simulink library "AEMS_Standard_Library"  (R2016b)
settings: Solver=ode45  StartTime=0.0  StopTime=10.0  RelTol=1e-3
undefined symbols (not defined in the file or in its folder): BkPY, carto, Cbx_extegr, Cbx_lpegrsys, Cbx_portegr, Cnx_bnk_nr_conf, Cnx_cyl_nr_conf, ConfigManagement, configuration_management, Cxx_dcm_io_tmr_end_xxxx, Cxx_dcm_rt_tmr_end, Cxx_DID_xxxx_IO_max, Cxx_DID_xxxx_IO_min, Cxx_egrhsofs, Cxx_vmaniegi, DEM_DEBOUNCE_FREEZE, DEM_DTR_CTL_INVISIBLE, DEM_DTR_CTL_NORMAL, Dem_DtrId2_XXX, Dem_DtrId3_XXX, Dem_DtrId4_XXX, Dem_DtrId5_XXX, Dem_DtrId6_XXX, Dem_DtrId7_XXX, Dem_DtrId8_XXX, Dem_DtrId9_XXX, Dem_DtrId_XXX, Dem_EnableConditionId2_XXX, Dem_EnableConditionId3_XXX, Dem_EnableConditionId4_XXX, Dem_EnableConditionId5_XXX, Dem_EnableConditionId6_XXX, Dem_EnableConditionId7_XXX, Dem_EnableConditionId8_XXX, Dem_EnableConditionId_XXX, Dem_EventId, Dem_EventId2_XXX, Dem_EventId3_XXX, Dem_EventId4_XXX, Dem_EventId5_XXX, Dem_EventId6_XXX, Dem_EventId7_XXX, Dem_EventId8_XXX, Dem_EventId9_XXX, Dem_EventId_Device_Faulttype, Dem_EventId_XXX, DEM_IUMPR_GENERAL_DENOMINATOR, DEM_OPCYC_IGNITION, Dem_RatioId2_XXX, Dem_RatioId3_XXX, Dem_RatioId4_XXX, Dem_RatioId5_XXX, Dem_RatioId6_XXX, Dem_RatioId7_XXX, Dem_RatioId8_XXX, Dem_RatioId_XXX, Dem_StorageConditionId2_XXX, Dem_StorageConditionId3_XXX, Dem_StorageConditionId4_XXX, Dem_StorageConditionId5_XXX ... (+65)
libraries: AEMS_Standard_Library x477, simulink x2
(part 15 of 39)

== system AEMS_Standard_Library/TIMER ==
  AEMS_SW_TIMER2 : Subsystem  Tag=[LIB]  mask(AEMS_SW_TIMER2){}
      mask help:
      | The block starts counter(Time) from zero when 'Start' input is
      | true and gets incremented in each time step with the 'Timestep'
      | value. The couter(Time) gets reset when 'Stop' becomes equal to true.
      settings: AttributesFormatString=%<MaskType>
      mask Help:
      | eval('path_lib=fileparts(which(''AEMS_Standard_Library''));');
      | doc_path = [path_lib '\help\AEMS_SW_TIMER2.pdf'];
      | eval('open(doc_path)')
      mask Display: disp(get_param(gcb,'name'));
  AEMS_SW_TIMER_INIT : Subsystem  Tag=[LIB]  mask(AEMS_SW_TIMER_INIT){}
      mask help: This block is a Software Timer. Increments the timer count with respect to given timestep. 'Init' input is to make the timer value initialized to 0.
      settings: AttributesFormatString=%<MaskType>
      mask Help:
      | eval('path_lib=fileparts(which(''AEMS_Standard_Library''));');
      | doc_path = [path_lib '\help\AEMS_SW_TIMER_INIT.pdf'];
      | eval('open(doc_path)')
      mask Display: disp('AEMS_SW_TIMER_INIT');
  AEMS_TIMER : Subsystem  Tag=[LIB]  mask(AEMS_TIMER){sample_time=0.01}
      mask prompts: sample_time "Clock :"
      mask help:
      | Timer
      |
      | I/O
      |  start_flag
      |    1 : timer count up
      |    0 : timer clear
      |  target_time
      |    Target time
      |
      |  alarm
      |    1 : timer_value >= target_time
      |    0 : timer_value < target_time
      |  timer_value
      |    Timer value(up count)
      mask init:
      | name=get_param(gcb,'MaskValueString');
      | sample_time=str2num(name);
      settings: AttributesFormatString="%<MaskType>\\nClock :  = %<sample_time>"
      mask Help:
      | eval('path_lib=fileparts(which(''AEMS_Standard_Library''));');
      | mskblk=get_param(gcbh,'MaskType');
      | doc_path = [path_lib '\help\',mskblk,'.pdf'];
      | eval('open(doc_path)');
      mask TypeOptions sample_time: 0.001 | 0.002 | 0.004 | 0.01 | 0.02 | 0.1
      mask Display: disp(sprintf('Clock = %s', char(name)))
  AEMS_TIMER1 : Subsystem  Tag=[LIB]  mask(AEMS_TIMER1){timeoutinit=0, initinit=0}
      mask prompts: timeoutinit "Timeout output initialisation"; initinit "Init input initialisation"
      mask help:
      | This block starts a timer and generates a timeout signal when the required duration has elapsed.The duration in seconds is set on edge rising init signal  and counting phase begins.Output timer gives the left time in seconds, that must pass before generating the timeout signal.If the init signal is true after the power supply, and if the timer must start, set init input initialisation to 0, else set it to 1.
      | If the timeout output must start at true, set timeout output initialisation to 1, else set it to 0.
      settings: AttributesFormatString=%<MaskType>\nTimeout output initialisation=%<timeoutinit>\nInit input initialisation=%<initinit>
      mask Help:
      | eval('path_lib=fileparts(which(''AEMS_Standard_Library''));');
      | doc_path = [path_lib '\help\AEMS_TIMER1.pdf'];
      | eval('open(doc_path)')
      mask Display:
      | plot([0.1 0.15 0.15 0.2 0.2 0.35],[0.67 0.67 0.9 0.9 0.67 0.67]);
      | plot([0.45 0.5 0.5 0.7 0.9],[0.05 0.05 0.3 0.05 0.05])
      | plot([0.45 0.7 0.7 0.9],[0.67 0.67 0.9 0.9])
  AEMS_TIMER_H : Subsystem  Tag=[LIB]  mask(AEMS_TIMER_H){sample_time=0.01}
      mask prompts: sample_time "Clock :"
      mask help:
      | Timer with holder
      |
      | I/O
      |  start_flag
      |    1 : timer count up
      |    0 : timer hold
      |  clear_flag
      |    1 : timer clear
      |    0 : None
      |  target_time
      |    Target time
      |
      |  alarm
      |    1 : timer_value >= target_time
      |    0 : timer_value < target_time
      |  timer_value
      |    Timer value(up count)
      mask init:
      | name=get_param(gcb,'MaskValueString');
      | sample_time=str2num(name);
      settings: AttributesFormatString="%<MaskType>\\nClock :  = %<sample_time>"
      mask Help:
      | eval('path_lib=fileparts(which(''AEMS_Standard_Library''));');
      | mskblk=get_param(gcbh,'MaskType');
      | doc_path = [path_lib '\help\',mskblk,'.pdf'];
      | eval('open(doc_path)');
      mask TypeOptions sample_time: 0.001 | 0.002 | 0.004 | 0.01 | 0.02 | 0.1
      mask Display: disp(sprintf('Clock = %s', char(name)))
  AEMS_TURN_OFF_DELAY : Subsystem  Tag=[LIB]  mask(AEMS_TURN_OFF_DELAY){timeoutinit=0, initinit=0}
      mask prompts: timeoutinit "Output initialization (0 or 1)"; initinit "Input initialization (0 or 1)"
      mask help:
      | When input is toggled from low to high, the output will respond immediately to the input by setting output low to high.
      | When input is toggled from high to low, the output will set from high to low after delaytime elapses.
      settings: AttributesFormatString=%<MaskType>\nOutput initialization=%<timeoutinit>\nInput initialization=%<initinit>
      mask Help:
      | eval('path_lib=fileparts(which(''AEMS_Standard_Library''));');
      | doc_path = [path_lib '\help\AEMS_TURN_OFF_DELAY.pdf'];
      | eval('open(doc_path)')
      mask Display: disp('AEMS_TURN_OFF_DELAY')
  AEMS_TURN_ON_DELAY : Subsystem  Tag=[LIB]  mask(AEMS_TURN_ON_DELAY){timeoutinit=0, initinit=0}
      mask prompts: timeoutinit "Output initialization (0 or 1)"; initinit "Input initialization (0 or 1)"
      mask help:
      | This block delays the output in rising edge state of output signal. The output (Out) is a boolean signal changes from 0 to 1 after the specified delay time.
      |
      | Initializations:
      | - Output initialization = beginning state of Output signal.
      | - Input initialization = state of Signal at -t used to determine the presence of a rising/falling edge at the first simulation step.
      settings: AttributesFormatString=%<MaskType>\nOutput initialization=%<timeoutinit>\nInput initialization=%<initinit>
      mask Help:
      | eval('path_lib=fileparts(which(''AEMS_Standard_Library''));');
      | doc_path = [path_lib '\help\AEMS_TURN_ON_DELAY.pdf'];
      | eval('open(doc_path)')
      mask Display:
      | plot([3 3.5 3.5 4 4 5 5 7.5 7.5 8.5], [5 5 6 6 5 5 6 6 5 5]);
      | plot([3 6.5 6.5 7.5 7.5 8.5], [2 2 3 3 2 2]);
      | plot([3 4.5], [5 6]);
      | plot([3 4.5], [6 5]);
      | text(5,0.4, 'Duration');
      | plot([5 6.5], [1 1]);
      | plot([5.2 5 5.2], [0.8 1 1.2]);
      | plot([6.3 6.5 6.3], [0.8 1 1.2]);
      | plot([5 5],[4.7 1.3]);
      | plot([6.5 6.5],[1.8 1.3]);
      | plot([7.5 7.5],[4.7 3.7]);
      | plot([0], [0]);
      | plot([8], [7]);

== system AEMS_Standard_Library/TRIGGER ==
  AEMS_EVENT : Subsystem  Tag=[LIB]  mask(AEMS_EVENT){sample_time=0.01, event_time=0.1}
      mask help:
      | Down edge event : Every Event_time
      |
      | * Can not use AEMS_EVENT library in triggered/enabled subsystem
      mask init:
      | name=get_param(gcb,'MaskValueString');
      | name=sprintf(strrep(name,'|','\n'));
      | name=strread(name,'%s','delimiter',',');
      settings: AttributesFormatString=%<MaskType>
      mask Help:
      | eval('path_lib=fileparts(which(''AEMS_Standard_Library''));');
      | mskblk=get_param(gcbh,'MaskType');
      | doc_path = [path_lib '\help\',mskblk,'.pdf'];
      | eval('open(doc_path)');
      mask Display: disp(sprintf('Sample_time = %s \nEvent_time = %s', char(name(1)) , char(name(2))))

== system AEMS_Standard_Library/BIT_OPERATION/AEMS_BITWISEAND ==
  In : Inport
  Mask : Inport  Port=2
  Chart : Stateflow chart
  Out : Outport
  wires:
  Chart/1(Out) -> Out/1
  Mask/1 -> Chart/2(Mask)
  In/1 -> Chart/1(Input_data)

== system AEMS_Standard_Library/BIT_OPERATION/AEMS_BITWISEOR ==
  In : Inport
  Mask : Inport  Port=2
  Chart : Stateflow chart
  Out : Outport
  wires:
  Chart/1(Out) -> Out/1
  Mask/1 -> Chart/2(Mask)
  In/1 -> Chart/1(Input_data)

== system AEMS_Standard_Library/BIT_OPERATION/AEMS_BITWISEXOR ==
  In : Inport
  Mask : Inport  Port=2
  Chart : Stateflow chart
  Out : Outport
  wires:
  In/1 -> Chart/1(Input_data)
  Mask/1 -> Chart/2(Mask)
  Chart/1(Out) -> Out/1

== system AEMS_Standard_Library/BIT_OPERATION/AEMS_BIT_GET ==
  In : Inport  Tag=AM,In,0,1,Name,C;CMP,Port,PortWidth,SampleTime;
  Bit_number : Inport  Tag=AM,In,0,1,Name,C;CMP,Port,PortWidth,SampleTime;  Port=2
  Chart : Stateflow chart  TreatAsAtomicUnit=on
  Bit_value : Outport  Tag=AM,Out,1,0,Name,NC;CMP,Port,OutputWhenDisabled,InitialOutput;
  wires:
  In/1 -> Chart/1(In)
  Chart/1(Bit_value) -> Bit_value/1
  Bit_number/1 -> Chart/2(Bit_number)

== system AEMS_Standard_Library/BIT_OPERATION/AEMS_BIT_SET16 ==
  Bit1 : Inport  Tag=AM,In,0,1,Name,C;CMP,Port,PortWidth,SampleTime;  OutDataTypeStr=boolean
  Bit2 : Inport  Tag=AM,In,0,1,Name,C;CMP,Port,PortWidth,SampleTime;  Port=2  OutDataTypeStr=boolean
  Bit3 : Inport  Tag=AM,In,0,1,Name,C;CMP,Port,PortWidth,SampleTime;  Port=3  OutDataTypeStr=boolean
  Bit4 : Inport  Tag=AM,In,0,1,Name,C;CMP,Port,PortWidth,SampleTime;  Port=4  OutDataTypeStr=boolean
  Bit5 : Inport  Tag=AM,In,0,1,Name,C;CMP,Port,PortWidth,SampleTime;  Port=5  OutDataTypeStr=boolean
  Bit6 : Inport  Tag=AM,In,0,1,Name,C;CMP,Port,PortWidth,SampleTime;  Port=6  OutDataTypeStr=boolean
  Bit7 : Inport  Tag=AM,In,0,1,Name,C;CMP,Port,PortWidth,SampleTime;  Port=7  OutDataTypeStr=boolean
  Bit8 : Inport  Tag=AM,In,0,1,Name,C;CMP,Port,PortWidth,SampleTime;  Port=8  OutDataTypeStr=boolean
  Bit9 : Inport  Tag=AM,In,0,1,Name,C;CMP,Port,PortWidth,SampleTime;  Port=9  OutDataTypeStr=boolean
  Bit10 : Inport  Tag=AM,In,0,1,Name,C;CMP,Port,PortWidth,SampleTime;  Port=10  OutDataTypeStr=boolean
  Bit11 : Inport  Tag=AM,In,0,1,Name,C;CMP,Port,PortWidth,SampleTime;  Port=11  OutDataTypeStr=boolean
  Bit12 : Inport  Tag=AM,In,0,1,Name,C;CMP,Port,PortWidth,SampleTime;  Port=12  OutDataTypeStr=boolean
  Bit13 : Inport  Tag=AM,In,0,1,Name,C;CMP,Port,PortWidth,SampleTime;  Port=13  OutDataTypeStr=boolean
  Bit14 : Inport  Tag=AM,In,0,1,Name,C;CMP,Port,PortWidth,SampleTime;  Port=14  OutDataTypeStr=boolean
  Bit15 : Inport  Tag=AM,In,0,1,Name,C;CMP,Port,PortWidth,SampleTime;  Port=15  OutDataTypeStr=boolean
  Bit16 : Inport  Tag=AM,In,0,1,Name,C;CMP,Port,PortWidth,SampleTime;  Port=16  OutDataTypeStr=boolean
  Chart : Stateflow chart  TreatAsAtomicUnit=on
  Out : Outport  Tag=AM,Out,1,0,Name,NC;CMP,Port,OutputWhenDisabled,InitialOutput;
  wires:
  Bit15/1 -> Chart/15(Bit15)
  Bit14/1 -> Chart/14(Bit14)
  Bit13/1 -> Chart/13(Bit13)
  Bit12/1 -> Chart/12(Bit12)
  Bit11/1 -> Chart/11(Bit11)
  Bit10/1 -> Chart/10(Bit10)
  Bit9/1 -> Chart/9(Bit9)
  Bit8/1 -> Chart/8(Bit8)
  Bit7/1 -> Chart/7(Bit7)
  Bit6/1 -> Chart/6(Bit6)
  Bit5/1 -> Chart/5(Bit5)
  Bit4/1 -> Chart/4(Bit4)
  Bit3/1 -> Chart/3(Bit3)
  Bit2/1 -> Chart/2(Bit2)
  Bit16/1 -> Chart/16(Bit16)
  Bit1/1 -> Chart/1(Bit1)
  Chart/1(Out) -> Out/1

== system AEMS_Standard_Library/BIT_OPERATION/AEMS_BIT_SET32 ==
  Bit1 : Inport  Tag=AM,In,0,1,Name,C;CMP,Port,PortWidth,SampleTime;  OutDataTypeStr=boolean
  Bit2 : Inport  Tag=AM,In,0,1,Name,C;CMP,Port,PortWidth,SampleTime;  Port=2  OutDataTypeStr=boolean
  Bit3 : Inport  Tag=AM,In,0,1,Name,C;CMP,Port,PortWidth,SampleTime;  Port=3  OutDataTypeStr=boolean
  Bit4 : Inport  Tag=AM,In,0,1,Name,C;CMP,Port,PortWidth,SampleTime;  Port=4  OutDataTypeStr=boolean
  Bit5 : Inport  Tag=AM,In,0,1,Name,C;CMP,Port,PortWidth,SampleTime;  Port=5  OutDataTypeStr=boolean
  Bit6 : Inport  Tag=AM,In,0,1,Name,C;CMP,Port,PortWidth,SampleTime;  Port=6  OutDataTypeStr=boolean
  Bit7 : Inport  Tag=AM,In,0,1,Name,C;CMP,Port,PortWidth,SampleTime;  Port=7  OutDataTypeStr=boolean
  Bit8 : Inport  Tag=AM,In,0,1,Name,C;CMP,Port,PortWidth,SampleTime;  Port=8  OutDataTypeStr=boolean
  Bit9 : Inport  Tag=AM,In,0,1,Name,C;CMP,Port,PortWidth,SampleTime;  Port=9  OutDataTypeStr=boolean
  Bit10 : Inport  Tag=AM,In,0,1,Name,C;CMP,Port,PortWidth,SampleTime;  Port=10  OutDataTypeStr=boolean
  Bit11 : Inport  Tag=AM,In,0,1,Name,C;CMP,Port,PortWidth,SampleTime;  Port=11  OutDataTypeStr=boolean
  Bit12 : Inport  Tag=AM,In,0,1,Name,C;CMP,Port,PortWidth,SampleTime;  Port=12  OutDataTypeStr=boolean
  Bit13 : Inport  Tag=AM,In,0,1,Name,C;CMP,Port,PortWidth,SampleTime;  Port=13  OutDataTypeStr=boolean
  Bit14 : Inport  Tag=AM,In,0,1,Name,C;CMP,Port,PortWidth,SampleTime;  Port=14  OutDataTypeStr=boolean
  Bit15 : Inport  Tag=AM,In,0,1,Name,C;CMP,Port,PortWidth,SampleTime;  Port=15  OutDataTypeStr=boolean
  Bit16 : Inport  Tag=AM,In,0,1,Name,C;CMP,Port,PortWidth,SampleTime;  Port=16  OutDataTypeStr=boolean
  Bit17 : Inport  Tag=AM,In,0,1,Name,C;CMP,Port,PortWidth,SampleTime;  Port=17  OutDataTypeStr=boolean
  Bit18 : Inport  Tag=AM,In,0,1,Name,C;CMP,Port,PortWidth,SampleTime;  Port=18  OutDataTypeStr=boolean
  Bit19 : Inport  Tag=AM,In,0,1,Name,C;CMP,Port,PortWidth,SampleTime;  Port=19  OutDataTypeStr=boolean
  Bit20 : Inport  Tag=AM,In,0,1,Name,C;CMP,Port,PortWidth,SampleTime;  Port=20  OutDataTypeStr=boolean
  Bit21 : Inport  Tag=AM,In,0,1,Name,C;CMP,Port,PortWidth,SampleTime;  Port=21  OutDataTypeStr=boolean
  Bit22 : Inport  Tag=AM,In,0,1,Name,C;CMP,Port,PortWidth,SampleTime;  Port=22  OutDataTypeStr=boolean
  Bit23 : Inport  Tag=AM,In,0,1,Name,C;CMP,Port,PortWidth,SampleTime;  Port=23  OutDataTypeStr=boolean
  Bit24 : Inport  Tag=AM,In,0,1,Name,C;CMP,Port,PortWidth,SampleTime;  Port=24  OutDataTypeStr=boolean
  Bit25 : Inport  Tag=AM,In,0,1,Name,C;CMP,Port,PortWidth,SampleTime;  Port=25  OutDataTypeStr=boolean
  Bit26 : Inport  Tag=AM,In,0,1,Name,C;CMP,Port,PortWidth,SampleTime;  Port=26  OutDataTypeStr=boolean
  Bit27 : Inport  Tag=AM,In,0,1,Name,C;CMP,Port,PortWidth,SampleTime;  Port=27  OutDataTypeStr=boolean
  Bit28 : Inport  Tag=AM,In,0,1,Name,C;CMP,Port,PortWidth,SampleTime;  Port=28  OutDataTypeStr=boolean
  Bit29 : Inport  Tag=AM,In,0,1,Name,C;CMP,Port,PortWidth,SampleTime;  Port=29  OutDataTypeStr=boolean
  Bit30 : Inport  Tag=AM,In,0,1,Name,C;CMP,Port,PortWidth,SampleTime;  Port=30  OutDataTypeStr=boolean
  Bit31 : Inport  Tag=AM,In,0,1,Name,C;CMP,Port,PortWidth,SampleTime;  Port=31  OutDataTypeStr=boolean
  Bit32 : Inport  Tag=AM,In,0,1,Name,C;CMP,Port,PortWidth,SampleTime;  Port=32  OutDataTypeStr=boolean
  Chart : Stateflow chart  TreatAsAtomicUnit=on
  Out : Outport  Tag=AM,Out,1,0,Name,NC;CMP,Port,OutputWhenDisabled,InitialOutput;  OutDataTypeStr=uint32
  wires:
  Bit15/1 -> Chart/15(Bit15)
  Bit14/1 -> Chart/14(Bit14)
  Bit13/1 -> Chart/13(Bit13)
  Bit12/1 -> Chart/12(Bit12)
  Bit11/1 -> Chart/11(Bit11)
  Bit10/1 -> Chart/10(Bit10)
  Bit9/1 -> Chart/9(Bit9)
  Bit8/1 -> Chart/8(Bit8)
  Bit7/1 -> Chart/7(Bit7)
  Bit6/1 -> Chart/6(Bit6)
  Bit5/1 -> Chart/5(Bit5)
  Bit4/1 -> Chart/4(Bit4)
  Bit3/1 -> Chart/3(Bit3)
  Bit2/1 -> Chart/2(Bit2)
  Bit16/1 -> Chart/16(Bit16)
  Bit1/1 -> Chart/1(Bit1)
  Chart/1(Out) -> Out/1
  Bit17/1 -> Chart/17(Bit17)
  Bit22/1 -> Chart/22(Bit22)
  Bit21/1 -> Chart/21(Bit21)
  Bit24/1 -> Chart/24(Bit24)
  Bit19/1 -> Chart/19(Bit19)
  Bit20/1 -> Chart/20(Bit20)
  Bit23/1 -> Chart/23(Bit23)
  Bit18/1 -> Chart/18(Bit18)
  Bit25/1 -> Chart/25(Bit25)
  Bit26/1 -> Chart/26(Bit26)
  Bit27/1 -> Chart/27(Bit27)
  Bit28/1 -> Chart/28(Bit28)
  Bit29/1 -> Chart/29(Bit29)
  Bit30/1 -> Chart/30(Bit30)
  Bit31/1 -> Chart/31(Bit31)
  Bit32/1 -> Chart/32(Bit32)

== system AEMS_Standard_Library/BIT_OPERATION/AEMS_BIT_SET8 ==
  Bit1 : Inport  Tag=AM,In,0,1,Name,C;CMP,Port,PortWidth,SampleTime;
  Bit2 : Inport  Tag=AM,In,0,1,Name,C;CMP,Port,PortWidth,SampleTime;  Port=2
  Bit3 : Inport  Tag=AM,In,0,1,Name,C;CMP,Port,PortWidth,SampleTime;  Port=3
  Bit4 : Inport  Tag=AM,In,0,1,Name,C;CMP,Port,PortWidth,SampleTime;  Port=4
  Bit5 : Inport  Tag=AM,In,0,1,Name,C;CMP,Port,PortWidth,SampleTime;  Port=5
  Bit6 : Inport  Tag=AM,In,0,1,Name,C;CMP,Port,PortWidth,SampleTime;  Port=6
  Bit7 : Inport  Tag=AM,In,0,1,Name,C;CMP,Port,PortWidth,SampleTime;  Port=7
  Bit8 : Inport  Tag=AM,In,0,1,Name,C;CMP,Port,PortWidth,SampleTime;  Port=8
  Chart : Stateflow chart  TreatAsAtomicUnit=on
  Out : Outport  Tag=AM,Out,1,0,Name,NC;CMP,Port,OutputWhenDisabled,InitialOutput;
  wires:
  Bit8/1 -> Chart/8(Bit8)
  Bit7/1 -> Chart/7(Bit7)
  Bit6/1 -> Chart/6(Bit6)
  Bit5/1 -> Chart/5(Bit5)
  Bit4/1 -> Chart/4(Bit4)
  Bit3/1 -> Chart/3(Bit3)
  Bit2/1 -> Chart/2(Bit2)
  Bit1/1 -> Chart/1(Bit1)
  Chart/1(Out) -> Out/1

== system AEMS_Standard_Library/BIT_OPERATION/AEMS_CONVERT_1BYTE_TO_2BYTE ==
  in_1byte_first : Inport  PortDimensions=1
      settings: AttributesFormatString=<tsample=%<SampleTime>>
  in_1byte_second : Inport  Port=2  PortDimensions=1
      settings: AttributesFormatString=<tsample=%<SampleTime>>
  AEMS_CONVERT_1BYTE_TO_8BIT : AEMS_Standard_Library/BIT_OPERATION/AEMS_CONVERT_1BYTE_TO_8BIT  Tag=[LIB]
  AEMS_CONVERT_1BYTE_TO_8BIT1 : AEMS_Standard_Library/BIT_OPERATION/AEMS_CONVERT_1BYTE_TO_8BIT  Tag=[LIB]
  CONVERT_16BIT_TO_2BYTE : Subsystem
  out_2byte : Outport
  wires:
  CONVERT_16BIT_TO_2BYTE/1(out_2byte) -> out_2byte/1  "out_2byte"
  in_1byte_second/1 -> AEMS_CONVERT_1BYTE_TO_8BIT/1  "in_1byte_second"
  in_1byte_first/1 -> AEMS_CONVERT_1BYTE_TO_8BIT1/1  "in_1byte_first"
  AEMS_CONVERT_1BYTE_TO_8BIT/8 -> CONVERT_16BIT_TO_2BYTE/16(bit15)
  AEMS_CONVERT_1BYTE_TO_8BIT/7 -> CONVERT_16BIT_TO_2BYTE/15(bit14)
  AEMS_CONVERT_1BYTE_TO_8BIT/6 -> CONVERT_16BIT_TO_2BYTE/14(bit13)
  AEMS_CONVERT_1BYTE_TO_8BIT/5 -> CONVERT_16BIT_TO_2BYTE/13(bit12)
  AEMS_CONVERT_1BYTE_TO_8BIT/4 -> CONVERT_16BIT_TO_2BYTE/12(bit11)
  AEMS_CONVERT_1BYTE_TO_8BIT/3 -> CONVERT_16BIT_TO_2BYTE/11(bit10)
  AEMS_CONVERT_1BYTE_TO_8BIT/2 -> CONVERT_16BIT_TO_2BYTE/10(bit9)
  AEMS_CONVERT_1BYTE_TO_8BIT/1 -> CONVERT_16BIT_TO_2BYTE/9(bit8)
  AEMS_CONVERT_1BYTE_TO_8BIT1/8 -> CONVERT_16BIT_TO_2BYTE/8(bit7)
  AEMS_CONVERT_1BYTE_TO_8BIT1/7 -> CONVERT_16BIT_TO_2BYTE/7(bit6)
  AEMS_CONVERT_1BYTE_TO_8BIT1/6 -> CONVERT_16BIT_TO_2BYTE/6(bit5)
  AEMS_CONVERT_1BYTE_TO_8BIT1/5 -> CONVERT_16BIT_TO_2BYTE/5(bit4)
  AEMS_CONVERT_1BYTE_TO_8BIT1/4 -> CONVERT_16BIT_TO_2BYTE/4(bit3)
  AEMS_CONVERT_1BYTE_TO_8BIT1/3 -> CONVERT_16BIT_TO_2BYTE/3(bit2)
  AEMS_CONVERT_1BYTE_TO_8BIT1/2 -> CONVERT_16BIT_TO_2BYTE/2(bit1)
  AEMS_CONVERT_1BYTE_TO_8BIT1/1 -> CONVERT_16BIT_TO_2BYTE/1(bit0)

== system AEMS_Standard_Library/BIT_OPERATION/AEMS_CONVERT_1BYTE_TO_8BIT ==
  in_1byte : Inport  OutDataTypeStr=uint8  PortDimensions=1
      settings: AttributesFormatString=<tsample=%<SampleTime>>
  Constant : Constant  Value=128  OutDataTypeStr=uint8
  Constant1 : Constant  Value=64  OutDataTypeStr=uint8
  Constant2 : Constant  Value=32  OutDataTypeStr=uint8
  Constant3 : Constant  Value=16  OutDataTypeStr=uint8
  Constant4 : Constant  Value=8  OutDataTypeStr=uint8
  Constant5 : Constant  Value=4  OutDataTypeStr=uint8
  Constant6 : Constant  Value=2  OutDataTypeStr=uint8
  Constant7 : Constant  OutDataTypeStr=uint8
  Relational Operator{,1..7} (8 alike) : RelationalOperator  OutDataTypeStr=boolean  RndMeth=Nearest  InputSameDT=on
  Sum{,1..6} (7 alike) : Sum  Inputs=-+  SaturateOnIntegerOverflow=on  InputSameDT=on
  Switch{,1..6} (7 alike) : Switch  Threshold=0.5  SaturateOnIntegerOverflow=on  InputSameDT=on
  bit0 : Outport
  bit1 : Outport  Port=2
  bit2 : Outport  Port=3
  bit3 : Outport  Port=4
  bit4 : Outport  Port=5
  bit5 : Outport  Port=6
  bit6 : Outport  Port=7
  bit7 : Outport  Port=8
  wires:
  Relational Operator7/1 -> bit0/1  "bit0"
  Switch6/1 -> Relational Operator7/1
  Constant7/1 -> Relational Operator7/2
  Switch5/1 -> Switch6/3, Sum6/2, Relational Operator6/1
  Relational Operator6/1 -> bit1/1, Switch6/2  "bit1"
  Sum6/1 -> Switch6/1
  Constant6/1 -> Relational Operator6/2, Sum6/1
  Switch4/1 -> Switch5/3, Sum5/2, Relational Operator5/1
  Relational Operator5/1 -> Switch5/2, bit2/1  "bit2"
  Sum5/1 -> Switch5/1
  Constant5/1 -> Sum5/1, Relational Operator5/2
  Switch3/1 -> Sum4/2, Switch4/3, Relational Operator4/1
  Relational Operator4/1 -> bit3/1, Switch4/2  "bit3"
  Sum4/1 -> Switch4/1
  Constant4/1 -> Relational Operator4/2, Sum4/1
  Switch2/1 -> Switch3/3, Sum3/2, Relational Operator3/1
  Relational Operator3/1 -> Switch3/2, bit4/1  "bit4"
  Sum3/1 -> Switch3/1
  Constant3/1 -> Sum3/1, Relational Operator3/2
  Switch1/1 -> Switch2/3, Sum2/2, Relational Operator2/1
  Relational Operator2/1 -> bit5/1, Switch2/2  "bit5"
  Sum2/1 -> Switch2/1
  Constant2/1 -> Relational Operator2/2, Sum2/1
  Relational Operator1/1 -> Switch1/2, bit6/1  "bit6"
  Sum1/1 -> Switch1/1
  Switch/1 -> Switch1/3, Sum1/2, Relational Operator1/1
  Constant1/1 -> Sum1/1, Relational Operator1/2
  Sum/1 -> Switch/1
  Relational Operator/1 -> Switch/2, bit7/1  "bit7"
  Constant/1 -> Sum/1, Relational Operator/2
  in_1byte/1 -> Switch/3, Sum/2, Relational Operator/1  "in_1byte"

== system AEMS_Standard_Library/BIT_OPERATION/AEMS_CONVERT_2BYTE_TO_1BYTE ==
  in_2byte : Inport  OutDataTypeStr=uint16  PortDimensions=1
      settings: AttributesFormatString=<tsample=%<SampleTime>>
  AEMS_CONVERT_8BIT_TO_1BYTE : AEMS_Standard_Library/BIT_OPERATION/AEMS_CONVERT_8BIT_TO_1BYTE  Tag=[LIB]
  AEMS_CONVERT_8BIT_TO_1BYTE1 : AEMS_Standard_Library/BIT_OPERATION/AEMS_CONVERT_8BIT_TO_1BYTE  Tag=[LIB]
  CONVERT_2BYTE_TO_16BIT : Subsystem
  out_1byte_first : Outport
  out_1byte_second : Outport  Port=2
  wires:
  AEMS_CONVERT_8BIT_TO_1BYTE/1 -> out_1byte_second/1  "out_1byte_second"
  AEMS_CONVERT_8BIT_TO_1BYTE1/1 -> out_1byte_first/1  "out_1byte_first"
  in_2byte/1 -> CONVERT_2BYTE_TO_16BIT/1(in_2byte)  "in_2byte"
  CONVERT_2BYTE_TO_16BIT/16(bit15) -> AEMS_CONVERT_8BIT_TO_1BYTE/8
  CONVERT_2BYTE_TO_16BIT/15(bit14) -> AEMS_CONVERT_8BIT_TO_1BYTE/7
  CONVERT_2BYTE_TO_16BIT/14(bit13) -> AEMS_CONVERT_8BIT_TO_1BYTE/6
  CONVERT_2BYTE_TO_16BIT/13(bit12) -> AEMS_CONVERT_8BIT_TO_1BYTE/5
  CONVERT_2BYTE_TO_16BIT/12(bit11) -> AEMS_CONVERT_8BIT_TO_1BYTE/4
  CONVERT_2BYTE_TO_16BIT/11(bit10) -> AEMS_CONVERT_8BIT_TO_1BYTE/3
  CONVERT_2BYTE_TO_16BIT/10(bit9) -> AEMS_CONVERT_8BIT_TO_1BYTE/2
  CONVERT_2BYTE_TO_16BIT/9(bit8) -> AEMS_CONVERT_8BIT_TO_1BYTE/1
  CONVERT_2BYTE_TO_16BIT/8(bit7) -> AEMS_CONVERT_8BIT_TO_1BYTE1/8
  CONVERT_2BYTE_TO_16BIT/7(bit6) -> AEMS_CONVERT_8BIT_TO_1BYTE1/7
  CONVERT_2BYTE_TO_16BIT/6(bit5) -> AEMS_CONVERT_8BIT_TO_1BYTE1/6
  CONVERT_2BYTE_TO_16BIT/5(bit4) -> AEMS_CONVERT_8BIT_TO_1BYTE1/5
  CONVERT_2BYTE_TO_16BIT/4(bit3) -> AEMS_CONVERT_8BIT_TO_1BYTE1/4
  CONVERT_2BYTE_TO_16BIT/3(bit2) -> AEMS_CONVERT_8BIT_TO_1BYTE1/3
  CONVERT_2BYTE_TO_16BIT/2(bit1) -> AEMS_CONVERT_8BIT_TO_1BYTE1/2
  CONVERT_2BYTE_TO_16BIT/1(bit0) -> AEMS_CONVERT_8BIT_TO_1BYTE1/1

== system AEMS_Standard_Library/BIT_OPERATION/AEMS_CONVERT_8BIT_TO_1BYTE ==
  bit0 : Inport  OutDataTypeStr=boolean  PortDimensions=1
      settings: AttributesFormatString=<tsample=%<SampleTime>>
  bit1 : Inport  Port=2  OutDataTypeStr=boolean  PortDimensions=1
      settings: AttributesFormatString=<tsample=%<SampleTime>>
  bit2 : Inport  Port=3  OutDataTypeStr=boolean  PortDimensions=1
      settings: AttributesFormatString=<tsample=%<SampleTime>>
  bit3 : Inport  Port=4  OutDataTypeStr=boolean  PortDimensions=1
      settings: AttributesFormatString=<tsample=%<SampleTime>>
  bit4 : Inport  Port=5  OutDataTypeStr=boolean  PortDimensions=1
      settings: AttributesFormatString=<tsample=%<SampleTime>>
  bit5 : Inport  Port=6  OutDataTypeStr=boolean  PortDimensions=1
      settings: AttributesFormatString=<tsample=%<SampleTime>>
  bit6 : Inport  Port=7  OutDataTypeStr=boolean  PortDimensions=1
      settings: AttributesFormatString=<tsample=%<SampleTime>>
  bit7 : Inport  Port=8  OutDataTypeStr=boolean  PortDimensions=1
      settings: AttributesFormatString=<tsample=%<SampleTime>>
  Constant : Constant  OutDataTypeStr=uint8
  Constant{1,3,5,7,9,11,13,15} (8 alike) : Constant  Value=0  OutDataTypeStr=uint8
  Constant10 : Constant  Value=32  OutDataTypeStr=uint8
  Constant12 : Constant  Value=64  OutDataTypeStr=uint8
  Constant14 : Constant  Value=128  OutDataTypeStr=uint8
  Constant2 : Constant  Value=2  OutDataTypeStr=uint8
  Constant4 : Constant  Value=4  OutDataTypeStr=uint8
  Constant6 : Constant  Value=8  OutDataTypeStr=uint8
  Constant8 : Constant  Value=16  OutDataTypeStr=uint8
  Sum : Sum  Inputs=++++++++  SaturateOnIntegerOverflow=on  InputSameDT=on
  Switch{,1..7} (8 alike) : Switch  Threshold=0.5  SaturateOnIntegerOverflow=on  InputSameDT=on
      settings: AttributesFormatString=<threshold=%<threshold>>
  out_1byte : Outport
  wires:
  Sum/1 -> out_1byte/1  "out_1byte"
  Switch7/1 -> Sum/8
  Switch6/1 -> Sum/7
  Switch5/1 -> Sum/6
  Switch4/1 -> Sum/5
  Switch3/1 -> Sum/4
  Switch2/1 -> Sum/3
  Switch1/1 -> Sum/2
  Switch/1 -> Sum/1
  Constant15/1 -> Switch7/3
  Constant14/1 -> Switch7/1
  bit7/1 -> Switch7/2  "bit7"
  Constant13/1 -> Switch6/3
  Constant12/1 -> Switch6/1
  bit6/1 -> Switch6/2  "bit6"
  Constant11/1 -> Switch5/3
  Constant10/1 -> Switch5/1
  bit5/1 -> Switch5/2  "bit5"
  Constant9/1 -> Switch4/3
  Constant8/1 -> Switch4/1
  bit4/1 -> Switch4/2  "bit4"
  Constant7/1 -> Switch3/3
  Constant6/1 -> Switch3/1
  bit3/1 -> Switch3/2  "bit3"
  Constant5/1 -> Switch2/3
  Constant4/1 -> Switch2/1
  bit2/1 -> Switch2/2  "bit2"
  Constant3/1 -> Switch1/3
  Constant2/1 -> Switch1/1
  bit1/1 -> Switch1/2  "bit1"
  Constant1/1 -> Switch/3
  Constant/1 -> Switch/1
  bit0/1 -> Switch/2  "bit0"

== system AEMS_Standard_Library/BIT_OPERATION/AEMS_CONVERT_TO_UNSIGNED_SI ==
  In : Inport
  Add : Sum  OutDataTypeStr=u_inp_data  SaturateOnIntegerOverflow=on  InputSameDT=on
      settings: AttributesFormatString=SAT = %<SaturateOnIntegerOverflow>
  Chart : Stateflow chart  TreatAsAtomicUnit=on
      settings: RTWSystemCode=Inline
  Constant0 : Constant  Value=0  OutDataTypeStr=inp_data
  MaskAllButSign : Constant  Value=MABS  OutDataTypeStr=inp_data
  MaskSign : Constant  Value=MS  OutDataTypeStr=u_inp_data
  Relational Operator : RelationalOperator  Operator=<  OutDataTypeStr=boolean  RndMeth=Simplest  InputSameDT=on
  Switch : Switch  Criteria=u2 ~= 0
      settings: AttributesFormatString=Criteria=%<Criteria>
  zerocst : Constant  Value=0  OutDataTypeStr=u_inp_data
  Out : Outport
  wires:
  Constant0/1 -> Relational Operator/2
  Relational Operator/1 -> Switch/2
  Switch/1 -> Add/1
  In/1 -> Chart/1(In), Relational Operator/1
  MaskSign/1 -> Switch/1
  Add/1 -> Out/1
  MaskAllButSign/1 -> Chart/2(Mask)
  Chart/1(Bit_value) -> Add/2
  zerocst/1 -> Switch/3

== system AEMS_Standard_Library/BIT_OPERATION/AEMS_EXTRACT_BIT ==
  In : Inport
  Chart : Stateflow chart  TreatAsAtomicUnit=on
      settings: RTWSystemCode=Inline
  Conversion : DataTypeConversion  RndMeth=Zero
  LHCst : Constant  Value=LH  OutDataTypeStr=u_inp_data
  RHCst : Constant  Value=RH  OutDataTypeStr=u_inp_data
  Bit_value : Outport
  wires:
  In/1 -> Chart/1(In)
  LHCst/1 -> Chart/2(Bit_number)
  Chart/1(Bit_value) -> Conversion/1
  RHCst/1 -> Chart/3(RH)
  Conversion/1 -> Bit_value/1

== system AEMS_Standard_Library/COM/AEMS_FRAME_SUPERVISION ==
  GADE : Inport
  Vbx_atsr_sys_ecu_ini_task10ms : Inport  Port=2
  rcpt_frm : Inport  Port=3
  Clear_Diag_Info : Inport  Port=4
  Frm_Detection_Cnd : Inport  Port=5
  Frm_Conf : Inport  Port=6
  Specific_Mon_Cnd : Inport  Port=7
  ECU_Category : Inport  Port=8
  JT1 : Inport  Port=9
  JT2 : Inport  Port=10
  TimeSched_dt : Inport  Port=11
  IgnitionSupplyConfirmation : Inport  Port=12
  BCM_Status : Inport  Port=13
  USM_Status : Inport  Port=14
  Dspl_Mask_Cnd : Inport  Port=15
  decM : Inport  Port=16
  decThres : Inport  Port=17
  VALMAX : Inport  Port=18
  M_Absent_ini : Inport  Port=19
  Unit Delay : UnitDelay  SampleTime=-1
      settings: AttributesFormatString=<initial=%<InitialCondition>>
  ecu_frm_detection : Subsystem
  ecu_frm_monitoring : Subsystem
  ecu_monitoring_display : Subsystem
  Frame_Detected : Outport
  Status : Outport  Port=2
  Diagnosis_Byte : Outport  Port=3
  M_Absent : Outport  Port=4
  wires:
  Unit Delay/1 -> ecu_frm_detection/4(Status_Loc2)
  M_Absent_ini/1 -> ecu_monitoring_display/6(M_Absent_ini)
  decM/1 -> ecu_monitoring_display/7(decM)
  decThres/1 -> ecu_monitoring_display/8(decThres)
  VALMAX/1 -> ecu_monitoring_display/9(VALMAX)
  Dspl_Mask_Cnd/1 -> ecu_monitoring_display/4(Dspl_Mask_Cnd)
  IgnitionSupplyConfirmation/1 -> ecu_frm_monitoring/7(IgnitionSupplyConfirmation), ecu_monitoring_display/3(IGN_Status)
  Clear_Diag_Info/1 -> ecu_frm_detection/1(Clear_Diag_Info), ecu_monitoring_display/2(ClearDiagInfo_dspl)
  rcpt_frm/1 -> ecu_monitoring_display/1(rcpt_frm_dspl), ecu_frm_monitoring/1(rcpt_frm)
  ecu_monitoring_display/1(Diagnosis_Byte) -> Diagnosis_Byte/1
  ecu_monitoring_display/2(M_Absent) -> M_Absent/1
  Vbx_atsr_sys_ecu_ini_task10ms/1 -> ecu_frm_monitoring/12(Vbx_atsr_sys_ecu_ini_task10ms), ecu_monitoring_display/11(Vbx_atsr_sys_ecu_ini_task10ms)
  ecu_frm_monitoring/2(Mon_Authorize) -> ecu_monitoring_display/10(Mon_Authorized)
  Specific_Mon_Cnd/1 -> ecu_frm_monitoring/8(Specific_Mon_Cnd)
  ECU_Category/1 -> ecu_frm_monitoring/6(ECU_Category)
  JT1/1 -> ecu_frm_monitoring/2(JT1)
  JT2/1 -> ecu_frm_monitoring/3(JT2)
  TimeSched_dt/1 -> ecu_frm_monitoring/4(TimeSched_dt)
  GADE/1 -> ecu_frm_monitoring/5(GADE)
  BCM_Status/1 -> ecu_frm_monitoring/10(BCM_Status)
  USM_Status/1 -> ecu_frm_monitoring/11(USM_Status)
  ecu_frm_detection/1(Frame_Detected) -> Frame_Detected/1, ecu_frm_monitoring/9(Frame_Detected)
  Frm_Detection_Cnd/1 -> ecu_frm_detection/2(Frm_Detection_Cnd)
  Frm_Conf/1 -> ecu_frm_detection/3(Frm_Conf)
  ecu_frm_monitoring/1(Status) -> Status/1, Unit Delay/1, ecu_monitoring_display/5(Status)

== system AEMS_Standard_Library/COM/AEMS_REQUEST_COUNTER ==
  note: Counts from lower to upper limit and resets back to lower
  Constant1 : Constant  OutDataTypeStr=InpType
  Constant4 : Constant  Value=0  OutDataTypeStr=Inherit: Inherit via back propagation
  DataTypeConversion : DataTypeConversion  OutDataTypeStr=InpConTyp  RndMeth=Zero
  RelationalOperator : RelationalOperator  Operator=<  OutDataTypeStr=boolean  RndMeth=Nearest  InputSameDT=on
  Sum4 : Sum  OutDataTypeStr=Inherit: Inherit via back propagation  RndMeth=Zero  SaturateOnIntegerOverflow=on  InputSameDT=on
      settings: AttributesFormatString=SAT = %<SaturateOnIntegerOverflow>
  Switch : Switch  Criteria=u2 ~= 0  RndMeth=Zero  InputSameDT=on
      settings: AttributesFormatString=Criteria=%<Criteria>
  UnitDelay : UnitDelay  SampleTime=-1
      settings: AttributesFormatString=<initial=%<InitialCondition>>
  Upper_Value : Constant  Value=253  OutDataTypeStr=Inherit: Inherit via back propagation
  Request_Number : Outport
  wires:
  Constant4/1 -> Switch/3
  UnitDelay/1 -> Sum4/1, RelationalOperator/1
  Sum4/1 -> Switch/1
  RelationalOperator/1 -> Switch/2
  Constant1/1 -> Sum4/2
  Switch/1 -> UnitDelay/1, DataTypeConversion/1
  Upper_Value/1 -> RelationalOperator/2
  DataTypeConversion/1 -> Request_Number/1

== system AEMS_Standard_Library/COM/AEMS_REQUEST_COUNTER_SWITCH ==
  note: We see here that it is just a test to see if the request number is different than from previous occurence.
      | If different, it means we have received (normally) one or many (shouldn't happen but better be prepared than nothing) write from Updated Value
      | Else we take the Output from Current Value
  Request_Number : Inport
  Current_Value : Constant  OutDataTypeStr=Inherit: Inherit via back propagation
  RelationalOperator : RelationalOperator  Operator===  OutDataTypeStr=boolean  RndMeth=Nearest  InputSameDT=on
  Switch : Switch  Criteria=u2 ~= 0  RndMeth=Zero  InputSameDT=on
      settings: AttributesFormatString=Criteria=%<Criteria>
  UnitDelay1 : UnitDelay  SampleTime=-1
      settings: AttributesFormatString=<initial=%<InitialCondition>>
  Updated_Value : Constant  OutDataTypeStr=Inherit: Inherit via back propagation
  Output : Outport
  wires:
  Current_Value/1 -> Switch/1
  Updated_Value/1 -> Switch/3
  RelationalOperator/1 -> Switch/2
  UnitDelay1/1 -> RelationalOperator/2
  Switch/1 -> Output/1
  Request_Number/1 -> RelationalOperator/1, UnitDelay1/1

== system AEMS_Standard_Library/COUNTER/AEMS_COUNTER ==
  start_flag : Inport  OutDataTypeStr=boolean
  clear_flag : Inport  Port=2  OutDataTypeStr=boolean
  Constant1 : Constant  OutDataTypeStr=uint8
  Constant2 : Constant  Value=0  OutDataTypeStr=uint8
  Constant3 : Constant  Value=limit_value  OutDataTypeStr=uint8
  Logical Operator : Logic  Operator=NOT  OutDataTypeStr=boolean
  MinMax : MinMax  Inputs=2  SaturateOnIntegerOverflow=on
  Sum1 : Sum  SaturateOnIntegerOverflow=on  InputSameDT=on
  Switch : Switch  Criteria=u2 ~= 0  SaturateOnIntegerOverflow=on
      settings: AttributesFormatString=Criteria=%<Criteria>
  Switch1 : Switch  Criteria=u2 ~= 0  SaturateOnIntegerOverflow=on
      settings: AttributesFormatString=Criteria=%<Criteria>
  Unit Delay : UnitDelay  SampleTime=-1
      settings: AttributesFormatString=<initial=%<InitialCondition>>
  count_value : Outport
  wires:
  Unit Delay/1 -> Switch/1, MinMax/2
  MinMax/1 -> Sum1/2
  Constant3/1 -> MinMax/1
  Constant2/1 -> Switch1/1
  Switch1/1 -> count_value/1, Unit Delay/1
  start_flag/1 -> Logical Operator/1
  clear_flag/1 -> Switch1/2
  Switch/1 -> Switch1/3
  Sum1/1 -> Switch/3
  Constant1/1 -> Sum1/1
  Logical Operator/1 -> Switch/2

== system AEMS_Standard_Library/DCM/AEMS_API_SUPPLIER_CALL ==
  In1 : Inport  OutDataTypeStr=uint8  PortDimensions=12
  In2 : Inport  Port=2  OutDataTypeStr=int16  PortDimensions=3
  Conv_Out1 : DataTypeConversion  SaturateOnIntegerOverflow=on  RndMeth=Zero
  G_Out1 : Ground
  T_In1 : Terminator
  T_In2 : Terminator
  Out1 : Outport  OutDataTypeStr=single  PortDimensions=1
  wires:
  In1/1 -> T_In1/1
  In2/1 -> T_In2/1
  Conv_Out1/1 -> Out1/1
  G_Out1/1 -> Conv_Out1/1

== system AEMS_Standard_Library/DCM/AEMS_APP_DID_WRITEDATA ==
  Value_DID_Write : Inport
  Request_Write_DID : Inport  Port=2
  Strategy : Inport  Port=3
  RelationalOperator : RelationalOperator  Operator=~=  OutDataTypeStr=boolean  RndMeth=Nearest  InputSameDT=on
  Switch : Switch  Criteria=u2 ~= 0  RndMeth=Zero  InputSameDT=on
      settings: AttributesFormatString=Criteria=%<Criteria>
  UnitDelay1 : UnitDelay  SampleTime=-1
      settings: AttributesFormatString=<initial=%<InitialCondition>>
  DID_Var : Outport
  wires:
  Request_Write_DID/1 -> UnitDelay1/1, RelationalOperator/1
  Switch/1 -> DID_Var/1
  UnitDelay1/1 -> RelationalOperator/2
  RelationalOperator/1 -> Switch/2
  Strategy/1 -> Switch/3
  Value_DID_Write/1 -> Switch/1

== system AEMS_Standard_Library/DCM/AEMS_APP_REQUEST_IOCONTROL ==
  Req_stadj_xxxx : Inport
  Req_rcecu_xxxx : Inport  Port=2
  Generic_Condition : Inport  Port=3
  Specific_Condition_xxxx : Inport  Port=4
  Value_Write_stadj_xxxx : Inport  Port=5
  Request_IOControl_Subsystem : Subsystem
  Timer_IOControl_Subsystem : Subsystem  TreatAsAtomicUnit=on
  Write_IOControl_Subsystem : Subsystem
  Flag_io_request_xxxx : Outport
  Flag_dcm_io_tmr_end_xxxx : Outport  Port=2
  Dcm_io_tmr_xxxx : Outport  Port=3
  Val_io_request_xxxx : Outport  Port=4
  wires:
  Req_stadj_xxxx/1 -> Timer_IOControl_Subsystem/1(Req_stadj_xxxx), Request_IOControl_Subsystem/1(Req_stadj_xxxx)
  Req_rcecu_xxxx/1 -> Request_IOControl_Subsystem/2(Req_rcecu_xxxx)
  Generic_Condition/1 -> Request_IOControl_Subsystem/3(Generic_Condition)
  Specific_Condition_xxxx/1 -> Request_IOControl_Subsystem/4(Specific_Condition_xxxx)
  Timer_IOControl_Subsystem/1(Req_tmr_end_xxxx) -> Request_IOControl_Subsystem/5(Req_tmr_end_xxxx)
  Request_IOControl_Subsystem/1(Flag_io_request_xxxx) -> Flag_io_request_xxxx/1
  Request_IOControl_Subsystem/2(Flag_dcm_io_tmr_end_xxxx) -> Flag_dcm_io_tmr_end_xxxx/1
  Timer_IOControl_Subsystem/2(Dcm_io_tmr_xxxx) -> Dcm_io_tmr_xxxx/1
  Value_Write_stadj_xxxx/1 -> Write_IOControl_Subsystem/1(Value_Write_stadj_xxxx)
  Write_IOControl_Subsystem/1(Val_io_request_xxxx) -> Val_io_request_xxxx/1

== system AEMS_Standard_Library/DCM/AEMS_APP_REQUEST_ROUTINE ==
  Req_sta_xxxx : Inport
  Req_stop_xxxx : Inport  Port=2
  Generic_Condition : Inport  Port=3
  Specific_Condition_xxxx : Inport  Port=4
  Request_Routine_Subsystem : Subsystem
  Timer_routine_Subsystem : Subsystem  TreatAsAtomicUnit=on
  Flag_sta_xxxx : Outport
  Flag_stop_xxxx : Outport  Port=2
  Flag_dcm_rt_tmr_end : Outport  Port=3
  Dcm_rt_tmr : Outport  Port=4
  wires:
  Request_Routine_Subsystem/3(Flag_dcm_rt_tmr_end) -> Flag_dcm_rt_tmr_end/1
  Timer_routine_Subsystem/1(Flag_req_tmr_end) -> Request_Routine_Subsystem/5(Flag_req_tmr_end)
  Timer_routine_Subsystem/2(Dcm_rt_tmr) -> Dcm_rt_tmr/1
  Request_Routine_Subsystem/2(Flag_stop_xxxx) -> Flag_stop_xxxx/1
  Request_Routine_Subsystem/1(Flag_sta_xxxx) -> Flag_sta_xxxx/1
  Specific_Condition_xxxx/1 -> Request_Routine_Subsystem/4(Specific_Condition_xxxx)
  Generic_Condition/1 -> Request_Routine_Subsystem/3(Generic_Condition)
  Req_stop_xxxx/1 -> Request_Routine_Subsystem/2(Req_stop_xxxx)
  Req_sta_xxxx/1 -> Request_Routine_Subsystem/1(Req_sta_xxxx), Timer_routine_Subsystem/1(Req_sta_xxxx)

== system AEMS_Standard_Library/DCM/AEMS_DCM_CLEARDIAGNOSTICINFORMATION ==
  Condition : Inport
  Callback_Subsystem : Subsystem
  ErrorCode : Terminator
  ErrorCode1 : Terminator
  flag_clr_req : Outport
  wires:
  Callback_Subsystem/1(flag_clr_req) -> flag_clr_req/1
  Callback_Subsystem/2(ErrorCode) -> ErrorCode/1  "ERRORCode"
  Callback_Subsystem/3(Std_ReturnType) -> ErrorCode1/1  "Std_ReturnType"
  Condition/1 -> Callback_Subsystem/1(Condition)  "condition"

== system AEMS_Standard_Library/DCM/AEMS_DCM_CONDITIONCHECKREAD ==
  note: CLIENT/SERVER:
      | Std_ReturnType Xxx_ConditionCheckRead(
      | Dcm_NegativeResponseCodeType* ErrorCode)
      |
      | ErrorCode in Terminator to inform this output to DCM Tool
  note: Routine_Status it's the status for all routines
  note: Vbx_cnd
  Condition_checkread : Inport
  Callback_Subsystem : Subsystem
  ErrorCode : Terminator
  ErrorCode1 : Terminator
  wires:
  Callback_Subsystem/2(Std_ReturnType) -> ErrorCode1/1  "Std_ReturnType"
  Callback_Subsystem/1(ErrorCode) -> ErrorCode/1  "ErrorCode"
  Condition_checkread/1 -> Callback_Subsystem/1(Condition_checkread)

== system AEMS_Standard_Library/DCM/AEMS_DCM_DID_READDATA ==
  Val_did_1 : Inport
  Callback_Subsystem : Subsystem
  Conversion_Subsystem : Subsystem
  Data : Terminator
  Std_ReturnType : Terminator
  wires:
  Callback_Subsystem/2(Std_ReturnType) -> Std_ReturnType/1  "Std_ReturnType"
  Callback_Subsystem/1(Data) -> Data/1  "Data"
  Conversion_Subsystem/1(Value_Read_xxxx_DCM) -> Callback_Subsystem/1(Value_Read_xxxx_DCM)
  Val_did_1/1 -> Conversion_Subsystem/1(DID_Variable_1)

== system AEMS_Standard_Library/DCM/AEMS_DCM_DID_WRITEDATA ==
  Generic_Conditions_Write : Inport
  Specific_Conditions_Write_xxxx : Inport  Port=2
  Callback_Subsystem : Subsystem
  Conversion_Subsystem : AEMS_Standard_Library/SUB/AEMS_CONVERT_BYTE_TO_FLP  Tag=[LIB]  Resol=1  offset=0  DID_Datatype=uint8
      settings: AttributesFormatString=%<MaskType>\nResolution = %<Resol>\nOffset = %<offset>\nDIDType = %<DID_DataType>
  Data Type Conversion1 : DataTypeConversion  OutDataTypeStr=uint8  RndMeth=Zero
  Data_Type_Conversion : DataTypeConversion
  Demux : Demux  Outputs=[1]
  ErrorCode : Terminator
  ErrorCode1 : Terminator
  Ground : Ground
  Permission_Subsystem : Subsystem
  Flag_Request_xxxx_DCM : Outport
  DID_1 : Outport  Port=2
  wires:
  Ground/1 -> Data Type Conversion1/1
  Callback_Subsystem/3(Std_ReturnType) -> ErrorCode1/1  "Std_ReturnType"
  Generic_Conditions_Write/1 -> Permission_Subsystem/1(Generic_conditions_Write)
  Specific_Conditions_Write_xxxx/1 -> Permission_Subsystem/2(Specific_conditions_Write_xxxx)
  Callback_Subsystem/1(Request_Write_xxxx_DCM) -> Flag_Request_xxxx_DCM/1
  Permission_Subsystem/1(Permission) -> Callback_Subsystem/1(Permission)  "Permission"
  Callback_Subsystem/2(ErrorCode) -> ErrorCode/1  "ErrorCode"
  Data Type Conversion1/1 -> Demux/1
  Conversion_Subsystem/1 -> Data_Type_Conversion/1
  Data_Type_Conversion/1 -> DID_1/1
  Demux/1 -> Conversion_Subsystem/1  "Data"

== system AEMS_Standard_Library/DCM/AEMS_DCM_GETDATA ==
  Convblock_Val_1 : DataTypeConversion  SaturateOnIntegerOverflow=on  RndMeth=Zero
  Convblock_Val_2 : DataTypeConversion  SaturateOnIntegerOverflow=on  RndMeth=Zero
  Data Type Conversion : DataTypeConversion  OutDataTypeStr=uint8
  Data Type Conversion1 : DataTypeConversion  OutDataTypeStr=uint8  RndMeth=Zero
  Demux : Demux  Outputs=2
  Ground : Ground
  Ground1 : Ground
  Terminator : Terminator
  Val_1 : Outport
  Val_2 : Outport  Port=2
  wires:
  Data Type Conversion/1 -> Terminator/1  "Std_ReturnType"
  Ground1/1 -> Data Type Conversion/1
  Data Type Conversion1/1 -> Demux/1
  Ground/1 -> Data Type Conversion1/1  "Data"
  Demux/1 -> Convblock_Val_1/1
  Convblock_Val_1/1 -> Val_1/1
  Demux/2 -> Convblock_Val_2/1
  Convblock_Val_2/1 -> Val_2/1

== system AEMS_Standard_Library/DCM/AEMS_DCM_GETPROGCONDITIONS ==
  Flag_request : Inport
  Callback_Subsystem : Subsystem
  ErrorCode : Terminator
  ErrorCode1 : Terminator
  wires:
  Flag_request/1 -> Callback_Subsystem/1(Flag_request)  "Flag_request"
  Callback_Subsystem/2(Dcm_EcuStartModeType) -> ErrorCode1/1  "Dcm_EcuStartModeType"
  Callback_Subsystem/1(ProgConditions) -> ErrorCode/1  "ProgConditions"

== system AEMS_Standard_Library/DCM/AEMS_DCM_GETSESCTRLTYPE ==
  Callback_Subsystem : Subsystem
  Ground1 : Ground
  Terminator : Terminator
  Data : Outport  OutDataTypeStr=uint8
  wires:
  Callback_Subsystem/1(Data) -> Data/1
  Callback_Subsystem/2(Std_ReturnType) -> Terminator/1
  Ground1/1 -> Callback_Subsystem/1(SesCtrlType)

== system AEMS_Standard_Library/DCM/AEMS_DCM_IO_RETURN_CONTROL_TO_ECU ==
  Callback_Subsystem : Subsystem
  ErrorCode : Terminator
  ErrorCode1 : Terminator
  Logical Operator : Logic  Operator=NOT  OutDataTypeStr=boolean
  Unit Delay : UnitDelay  SampleTime=-1
      settings: AttributesFormatString=<initial=%<InitialCondition>>
  Flag_Req_RtCtrToECU : Outport
  wires:
  Callback_Subsystem/2(Std_ReturnType) -> ErrorCode1/1  "Std_ReturnType"
  Logical Operator/1 -> Flag_Req_RtCtrToECU/1, Unit Delay/1
  Unit Delay/1 -> Logical Operator/1
  Callback_Subsystem/1(ErrorCode) -> ErrorCode/1  "ErrorCode"

== system AEMS_Standard_Library/DCM/AEMS_DCM_IO_SHORT_TERM_ADJUSTMENT ==
  Generic_Conditions_RoutineIO : Inport
  Specific_Conditions_IO_XXXX : Inport  Port=2
  Callback_Subsystem : Subsystem
  Conversion_Subsystem : Subsystem
  ErrorCode : Terminator
  ErrorCode1 : Terminator
  Ground : Ground
  Permission_Subsystem : Subsystem
  Value_Write_xxxx_DCM : Outport
  Flag_Request_xxxx_DCM : Outport  Port=2
  wires:
  Callback_Subsystem/3(ErrorCode) -> ErrorCode/1  "ErrorCode"
  Callback_Subsystem/1(Value_Write_xxxx_DCM) -> Value_Write_xxxx_DCM/1
  Conversion_Subsystem/1(ControlStateInfo_flp) -> Callback_Subsystem/2(ControlStateInfo_flp)
  Ground/1 -> Conversion_Subsystem/1(ControlStateInfo)
  Callback_Subsystem/2(ShortTermAdjustement_flag_Request_xxxx_DCM) -> Flag_Request_xxxx_DCM/1
  Permission_Subsystem/1(Permission) -> Callback_Subsystem/1(Permission)
  Generic_Conditions_RoutineIO/1 -> Permission_Subsystem/1(Generic_Conditions_RoutineIO)
  Specific_Conditions_IO_XXXX/1 -> Permission_Subsystem/2(Specific_Conditions_IO_XXXX)
  Callback_Subsystem/4(Std_ReturnType) -> ErrorCode1/1  "Std_ReturnType"

== system AEMS_Standard_Library/DCM/AEMS_DCM_REQUEST_RESULT ==
  note: CLIENT/SERVER:
      | Std_ReturnType Xxx_RequestResults(DcmDspRoutineSignalType* dataOut_1,
      | Dcm_NegativeResponseCodeType* ErrorCode)
      |
      | dataOut_1 in Terminator to inform this output to DCM Tool
      | ErrorCode in Terminator to inform this output to DCM Tool
  Routine_xxxx_Status : Inport
  Callback_Subsystem : Subsystem
  ErrorCode : Terminator
  ErrorCode1 : Terminator
  dataOut_1 : Terminator
  wires:
  Routine_xxxx_Status/1 -> Callback_Subsystem/1(Routine_xxxx_Status)
  Callback_Subsystem/1(dataOut_1) -> dataOut_1/1  "dataOut_1"
  Callback_Subsystem/2(ErrorCode) -> ErrorCode/1  "ErrorCode"
  Callback_Subsystem/3(Std_ReturnType) -> ErrorCode1/1  "Std_ReturnType"

== system AEMS_Standard_Library/DCM/AEMS_DCM_START_ROUTINE ==
  note: Routine_Status it's the status for all routine
      | Routines_xxxx_status it's a boolean to indicate if this routine is running or not
  note: CLIENT/SERVER:
      | Std_ReturnType Xxx_Start(DcmDspRoutineSignalType dataOut_1,
      | Dcm_NegativeResponseCodeType* ErrorCode)
      |
      | dataOut_1 in Terminator to inform this output to DCM Tool
      | ErrorCode in Terminator to inform this output to DCM Tool
  Generic_Conditions_Routine : Inport
  Specific_Conditions_Routine_xxxx : Inport  Port=2
  Routine_Status : Inport  Port=3
  Routine_xxxx_Status : Inport  Port=4
  Callback_Subsystem : Subsystem
  Constant : Constant  Value=0  OutDataTypeStr=uint8
  ErrorCode : Terminator
  ErrorCode1 : Terminator
  Permission_Subsystem : Subsystem
  dataOut_1 : Terminator
  Flag_request_xxxx_DCM : Outport
  wires:
  Generic_Conditions_Routine/1 -> Permission_Subsystem/1(Generic_Conditions_Routine)
  Specific_Conditions_Routine_xxxx/1 -> Permission_Subsystem/2(Specific_Conditions_Routine_xxxx)
  Permission_Subsystem/1(Permission) -> Callback_Subsystem/1(Permission)
  Callback_Subsystem/1(Flag_request_xxxx_DCM) -> Flag_request_xxxx_DCM/1
  Routine_Status/1 -> Permission_Subsystem/3(Routine_Status), Callback_Subsystem/2(Routine_Status)
  Routine_xxxx_Status/1 -> Callback_Subsystem/3(Routine_xxxx_Status)
  Callback_Subsystem/2(dataOut_1) -> dataOut_1/1  "dataOut_1"
  Callback_Subsystem/3(ErrorCode) -> ErrorCode/1  "ErrorCode"
  Constant/1 -> Callback_Subsystem/4(OpStatus)  "OpStatus"
  Callback_Subsystem/4(Std_ReturnType) -> ErrorCode1/1  "Std_ReturnType"

== system AEMS_Standard_Library/DCM/AEMS_DCM_STOP_ROUTINE ==
  note: CLIENT/SERVER:
      | Std_ReturnType Xxx_Stop(
      | DcmDspRoutineSignalType dataOut_1,
      | Dcm_NegativeResponseCodeType* ErrorCode
      | )
      | dataOut_1 in Terminator to inform this output to DCM Tool
      | ErrorCode in Terminator to inform this output to DCM Tool
  Routine_xxxx_Status : Inport
  Constant : Constant  Value=0  OutDataTypeStr=uint8
  ErrorCode : Terminator
  ErrorCode1 : Terminator
  Xxx_Stop_Callback : Subsystem
  dataOut_1 : Terminator
  Flag_request_xxxx_DCM : Outport  InitialOutput=0
  wires:
  Xxx_Stop_Callback/3(ErrorCode) -> ErrorCode/1  "ErrorCode"
  Xxx_Stop_Callback/2(dataOut_1) -> dataOut_1/1  "dataOut_1"
  Xxx_Stop_Callback/1(Flag_request_XXXX_DCM_Stop) -> Flag_request_xxxx_DCM/1
  Routine_xxxx_Status/1 -> Xxx_Stop_Callback/1(Routine_xxxx_Status)
  Xxx_Stop_Callback/4(Std_ReturnType) -> ErrorCode1/1  "Std_ReturnType"
  Constant/1 -> Xxx_Stop_Callback/2(OpStatus)  "OpStatus"

== system AEMS_Standard_Library/DCM/AEMS_FLOAT_TO_FXP ==
  phys : Inport  PortDimensions=1
      settings: AttributesFormatString=<tsample=%<SampleTime>>
  Constant : Constant  Value=Offset  OutDataTypeStr=Inherit: Inherit via back propagation
  Constant1 : Constant  Value=Resol  OutDataTypeStr=Inherit: Inherit via back propagation
  OutputDatatype : DataTypeConversion  OutDataTypeStr=uint8  SaturateOnIntegerOverflow=on  RndMeth=Zero
  Product : Product  Inputs=*/  OutDataTypeStr=Inherit: Inherit via back propagation  SaturateOnIntegerOverflow=on  RndMeth=Zero  InputSameDT=on
      settings: AttributesFormatString=SAT = %<SaturateOnIntegerOverflow>
  Sum : Sum  Inputs=+-  OutDataTypeStr=Inherit: Inherit via back propagation  RndMeth=Zero  SaturateOnIntegerOverflow=on  InputSameDT=on
      settings: AttributesFormatString=SAT = %<SaturateOnIntegerOverflow>
  fxp : Outport
  wires:
  OutputDatatype/1 -> fxp/1
  phys/1 -> Sum/1
  Sum/1 -> Product/1
  Constant1/1 -> Product/2
  Constant/1 -> Sum/2
  Product/1 -> OutputDatatype/1

== system AEMS_Standard_Library/DCM/AEMS_FLOAT_TO_FXP_WITH_LIMIT ==
  phys : Inport  PortDimensions=1
      settings: AttributesFormatString=<tsample=%<SampleTime>>
  Constant : Constant  Value=Offset  OutDataTypeStr=Inherit: Inherit via back propagation
  Constant1 : Constant  Value=Resol  OutDataTypeStr=Inherit: Inherit via back propagation
  Constant2 : Constant  Value=Min  OutDataTypeStr=Inherit: Inherit via back propagation
  Constant4 : Constant  Value=Max  OutDataTypeStr=Inherit: Inherit via back propagation
  MinMax : MinMax  Function=max  Inputs=2
  MinMax1 : MinMax  Inputs=2
  OutputDatatype : DataTypeConversion  OutDataTypeStr=uint8  SaturateOnIntegerOverflow=on  RndMeth=Zero
  Product : Product  Inputs=*/  OutDataTypeStr=Inherit: Inherit via back propagation  SaturateOnIntegerOverflow=on  RndMeth=Zero  InputSameDT=on
      settings: AttributesFormatString=SAT = %<SaturateOnIntegerOverflow>
  Sum : Sum  Inputs=+-  OutDataTypeStr=Inherit: Inherit via back propagation  RndMeth=Zero  SaturateOnIntegerOverflow=on  InputSameDT=on
      settings: AttributesFormatString=SAT = %<SaturateOnIntegerOverflow>
  fxp : Outport
  wires:
  Product/1 -> OutputDatatype/1
  Constant/1 -> Sum/2
  Constant1/1 -> Product/2
  Sum/1 -> Product/1
  OutputDatatype/1 -> fxp/1
  phys/1 -> MinMax/1
  MinMax1/1 -> Sum/1
  MinMax/1 -> MinMax1/2
  Constant2/1 -> MinMax/2
  Constant4/1 -> MinMax1/1
